simulink model "VariableGainControllerChangingParameters"  (R2018a)
settings: Solver=VariableStepAuto  StartTime=0.0  StopTime=10.0  RelTol=1e-3
libraries: simulink x6
settings Model: Creator=Dell  LastModifiedBy=Dell

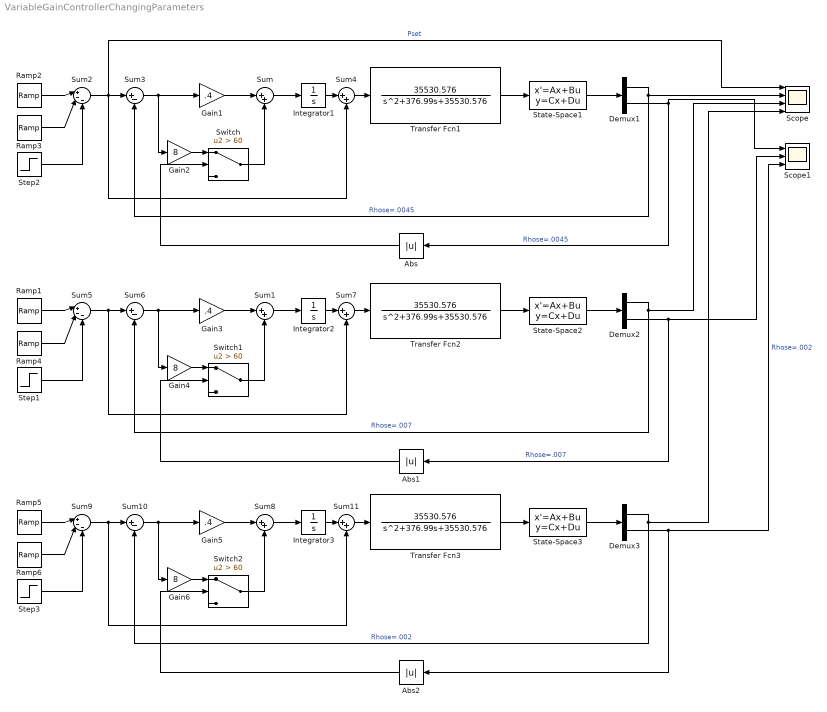
== system VariableGainControllerChangingParameters ==
  Abs : Abs
  Abs1 : Abs
  Abs2 : Abs
  Demux1 : Demux  Outputs=2
  Demux2 : Demux  Outputs=2
  Demux3 : Demux  Outputs=2
  Gain1 : Gain  Gain=.4
  Gain2 : Gain  Gain=8
  Gain3 : Gain  Gain=.4
  Gain4 : Gain  Gain=8
  Gain5 : Gain  Gain=.4
  Gain6 : Gain  Gain=8
  Integrator1 : Integrator
  Integrator2 : Integrator
  Integrator3 : Integrator
  Ramp1 : simulink/Sources/Ramp  slope=150  start=1  InitialOutput=5
  Ramp2 : simulink/Sources/Ramp  slope=150  start=1  InitialOutput=5
  Ramp3 : simulink/Sources/Ramp  slope=150  start=1.1  InitialOutput=0
  Ramp4 : simulink/Sources/Ramp  slope=150  start=1.1  InitialOutput=0
  Ramp5 : simulink/Sources/Ramp  slope=150  start=1  InitialOutput=5
  Ramp6 : simulink/Sources/Ramp  slope=150  start=1.1  InitialOutput=0
  Scope : Scope  NumInputPorts=4
  Scope1 : Scope  NumInputPorts=3
  State-Space1 : StateSpace  A=-5.443  B=5.063  C=[0.4557;-108.86]  D=[0.5063;101.266]  InitialCondition=0
  State-Space2 : StateSpace  A=-4.4371  B=3.9735  C=[0.5563;-88.7417]  D=[0.3974;79.4702]  InitialCondition=0
  State-Space3 : StateSpace  A=-7.2093  B=6.9767  C=[0.2791;-144.1860]  D=[0.6977;139.5349]  InitialCondition=0
  Step1 : Step  Time=5  After=15  SampleTime=0
  Step2 : Step  Time=5  After=15  SampleTime=0
  Step3 : Step  Time=5  After=15  SampleTime=0
  Sum{,1,4,7..8,11} (6 alike) : Sum  Inputs=|++
  Sum10 : Sum  Inputs=|+-
  Sum2 : Sum  Inputs=|+--
  Sum3 : Sum  Inputs=|+-
  Sum5 : Sum  Inputs=|+--
  Sum6 : Sum  Inputs=|+-
  Sum9 : Sum  Inputs=|+--
  Switch : Switch  Criteria=u2 > Threshold  Threshold=60
  Switch1 : Switch  Criteria=u2 > Threshold  Threshold=60
  Switch2 : Switch  Criteria=u2 > Threshold  Threshold=60
  Transfer Fcn1 : TransferFcn  Numerator=[35530.576]  Denominator=[1 376.99 35530.576]
  Transfer Fcn2 : TransferFcn  Numerator=[35530.576]  Denominator=[1 376.99 35530.576]
  Transfer Fcn3 : TransferFcn  Numerator=[35530.576]  Denominator=[1 376.99 35530.576]
  wires:
  Switch1/1 -> Sum1/2
  Ramp1/1 -> Sum5/1
  Abs1/1 -> Switch1/2
  Gain4/1 -> Switch1/1
  Sum1/1 -> Integrator2/1
  Ramp6/1 -> Sum9/2
  Gain3/1 -> Sum1/1
  Sum7/1 -> Transfer Fcn2/1
  Sum4/1 -> Transfer Fcn1/1
  Sum/1 -> Integrator1/1
  Abs/1 -> Switch/2
  Transfer Fcn1/1 -> State-Space1/1
  Sum3/1 -> Gain2/1, Gain1/1
  Step2/1 -> Sum2/3
  Sum6/1 -> Gain4/1, Gain3/1
  State-Space1/1 -> Demux1/1
  Gain5/1 -> Sum8/1
  Abs2/1 -> Switch2/2
  Step3/1 -> Sum9/3
  Demux1/1 -> Scope/2, Sum3/2  "Rhose=.0045"
  Sum8/1 -> Integrator3/1
  Sum2/1 -> Scope/1, Sum3/1, Sum4/2  "Pset"
  State-Space3/1 -> Demux3/1
  Switch/1 -> Sum/2
  Ramp5/1 -> Sum9/1
  State-Space2/1 -> Demux2/1
  Ramp3/1 -> Sum2/2
  Gain2/1 -> Switch/1
  Sum9/1 -> Sum10/1, Sum11/2
  Switch2/1 -> Sum8/2
  Transfer Fcn3/1 -> State-Space3/1
  Sum5/1 -> Sum6/1, Sum7/2
  Gain6/1 -> Switch2/1
  Ramp2/1 -> Sum2/1
  Gain1/1 -> Sum/1
  Integrator3/1 -> Sum11/1
  Integrator2/1 -> Sum7/1
  Sum10/1 -> Gain6/1, Gain5/1
  Ramp4/1 -> Sum5/2
  Integrator1/1 -> Sum4/1
  Demux1/2 -> Scope1/1, Abs/1  "Rhose=.0045"
  Demux2/1 -> Scope/3, Sum6/2  "Rhose=.007"
  Sum11/1 -> Transfer Fcn3/1
  Transfer Fcn2/1 -> State-Space2/1
  Demux3/1 -> Scope/4, Sum10/2  "Rhose=.002"
  Demux2/2 -> Scope1/2, Abs1/1  "Rhose=.007"
  Demux3/2 -> Scope1/3, Abs2/1  "Rhose=.002"
  Step1/1 -> Sum5/3
